simulink model "makeOcT_th"  (R2020a)
settings: Solver=VariableStepAuto  StartTime=0.0  StopTime=0  RelTol=1e-3
libraries: makeOcT_cl x1
settings Model: Creator=Ayaz  LastModifiedBy=Ayaz

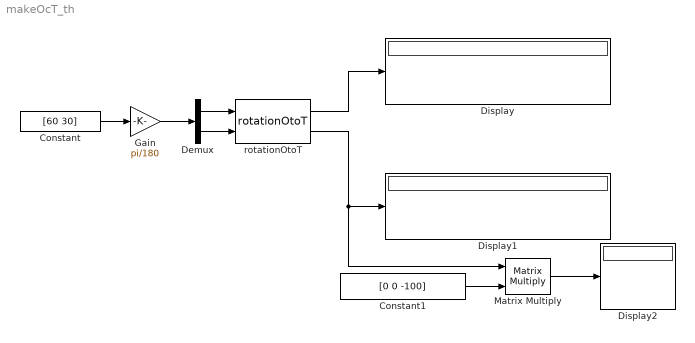
== system makeOcT_th ==
  Constant : Constant  Value=[60 30]
  Constant1 : Constant  Value=[0 0 -100]
  Demux : Demux  Outputs=2
  Display : Display
  Display1 : Display
  Display2 : Display
  Gain : Gain  Gain=pi/180
  Matrix Multiply : Product  Multiplication=Matrix(*)
  rotationOtoT : makeOcT_cl/rotationOtoT  SystemSampleTime=-1  Latency=0  AutoFrameSizeCalculation=off
  wires:
  rotationOtoT/1 -> Display/1
  rotationOtoT/2 -> Matrix Multiply/1, Display1/1
  Demux/1 -> rotationOtoT/1
  Demux/2 -> rotationOtoT/2
  Constant/1 -> Gain/1
  Gain/1 -> Demux/1
  Constant1/1 -> Matrix Multiply/2
  Matrix Multiply/1 -> Display2/1
